simulink model "motorControlRight"  (R2024b)
settings: Solver=VariableStepAuto  StartTime=0.0  StopTime=3  RelTol=1e-3
model workspace (MAT data in the model file):
  K = Simulink.Parameter
  K.Value = 4.2
  K.Complexity = 'real'
  K.Dimensions = [1 1]
  K.DataType = 'auto'
  Kp = 5
values from neighbouring files (symbols this model uses):
  K = 4.12    [runControlSimRight.m]    (also in runmotorsim.m = 2.2; runmotorsim2.m; runmotorsimRight.m)
  sigma = 14    [runControlSimRight.m]    (also in runmotorsim.m = 5; runmotorsim2.m; runmotorsimRight.m)
libraries: simulink x1
settings Model: Creator=bensmithva  LastModifiedBy=bensmithva

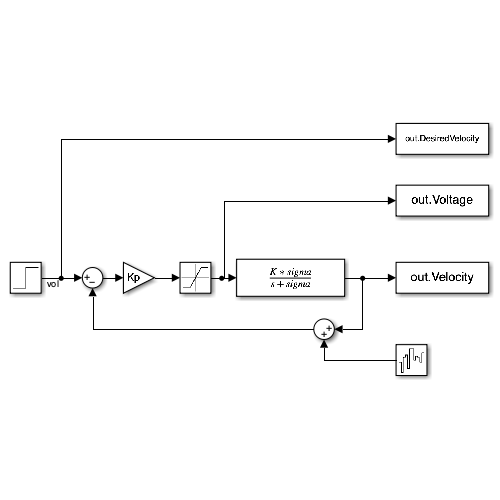
[thumbnail: Simulink's stored preview of the top-level diagram]
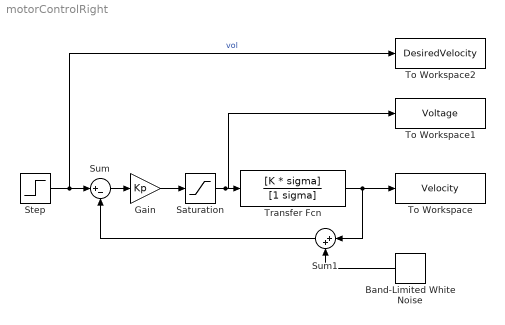
== system motorControlRight ==
  Band-Limited White Noise : simulink/Sources/Band-Limited White Noise  Cov=[0.0001]  Ts=0.01  seed=[23341]
  Gain : Gain  Gain=Kp
  Saturation : Saturate  UpperLimit=7.5  LowerLimit=-7.5
  Step : Step  After=10  SampleTime=0
  Sum : Sum  Inputs=|+-
  Sum1 : Sum  Inputs=|++
  To Workspace : ToWorkspace  VariableName=Velocity  SaveFormat=Timeseries  SampleTime=-1
  To Workspace1 : ToWorkspace  VariableName=Voltage  SaveFormat=Timeseries  SampleTime=-1
  To Workspace2 : ToWorkspace  VariableName=DesiredVelocity  SaveFormat=Timeseries  SampleTime=-1
  Transfer Fcn : TransferFcn  Numerator=[K * sigma]  Denominator=[1 sigma]
  wires:
  Transfer Fcn/1 -> Sum1/1, To Workspace/1
  Step/1 -> To Workspace2/1, Sum/1  "vol"
  Saturation/1 -> To Workspace1/1, Transfer Fcn/1
  Band-Limited White Noise/1 -> Sum1/2
  Sum1/1 -> Sum/2
  Sum/1 -> Gain/1
  Gain/1 -> Saturation/1
